simulink model "cascade"  (R2020b)
settings: Solver=VariableStepAuto  StartTime=0.0  StopTime=5  RelTol=1e-3
libraries: simulink x1
settings Model: Creator=Admin  LastModifiedBy=Admin

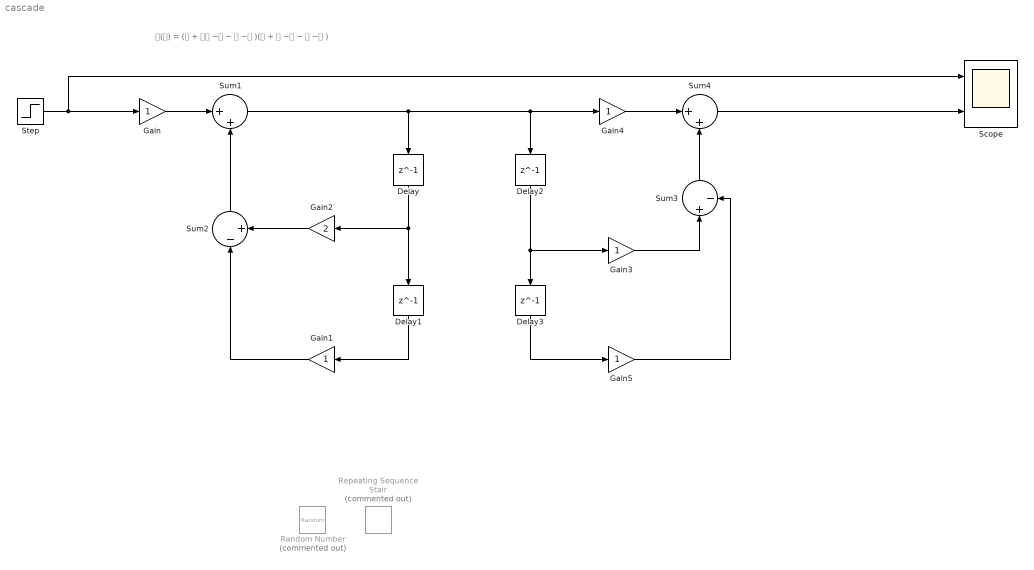
== system cascade ==
  note: 𝐇(𝐳) = (𝟏 + 𝟐𝐳 −𝟏 − 𝐳 −𝟐 )(𝟏 + 𝐳 −𝟏 − 𝐳 −𝟐 )
  Delay{,1..3} (4 alike) : Delay  DelayLength=1  InitialCondition=0
  Gain{,1,3..5} (5 alike) : Gain
  Gain2 : Gain  Gain=2
  Random Number : RandomNumber  Commented=on  SampleTime=0.1
  Repeating Sequence Stair : simulink/Sources/Repeating Sequence Stair  Commented=on  OutValues=[0 1 0 ].'  tsamp=-1  OutMin=[]  OutMax=[]  OutDataTypeStr=double  OutputDataTypeScalingMode=double  OutDataType=fixdt(0,8)  ConRadixGroup=Best Precision: Vector-wise  OutScaling=2^-12
  Scope : Scope  NumInputPorts=2
  Step : Step  SampleTime=0
  Sum1 : Sum  Inputs=|++
  Sum2 : Sum  Inputs=|-+
  Sum3 : Sum  Inputs=|+-
  Sum4 : Sum  Inputs=|++
  wires:
  Sum1/1 -> Gain4/1, Delay2/1, Delay/1
  Delay1/1 -> Gain1/1
  Gain1/1 -> Sum2/1
  Delay3/1 -> Gain5/1
  Delay/1 -> Delay1/1, Gain2/1
  Gain/1 -> Sum1/1
  Gain2/1 -> Sum2/2
  Sum2/1 -> Sum1/2
  Step/1 -> Scope/1, Gain/1
  Delay2/1 -> Gain3/1, Delay3/1
  Gain3/1 -> Sum3/1
  Gain5/1 -> Sum3/2
  Sum3/1 -> Sum4/2
  Gain4/1 -> Sum4/1
  Sum4/1 -> Scope/2
